simulink model "zad3_sim"  (R2014b)
settings: Solver=ode45  StartTime=0.0  StopTime=70  MaxStep=10  RelTol=1e-3
values from neighbouring files (symbols this model uses):
  a1 = -0.28    [set_params.m]
  a2 = -0.9    [set_params.m]
  a3 = 0.35    [set_params.m]
  a4 = 0.3    [set_params.m]
  K = 4.5    [set_params.m]
  T1 = 5    [set_params.m]
  T2 = 8    [set_params.m]
  Tp = 1    [zad10.m]    (also in zad11.m; zad3.m = Tp_vect(i); zad9.m)
settings Model: Creator=kuba  LastModifiedBy=kuba
settings DebuggingCC: SolverPrmCheckMsg=none

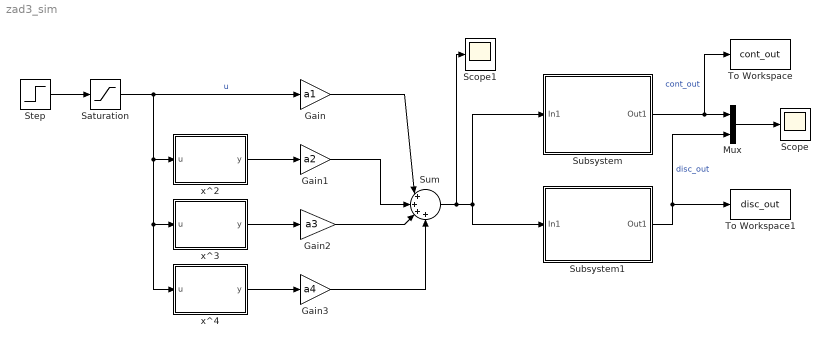
== system zad3_sim ==
  Gain : Gain  Gain=a1
  Gain1 : Gain  Gain=a2
  Gain2 : Gain  Gain=a3
  Gain3 : Gain  Gain=a4
  Mux : Mux  Inputs=2
  Saturation : Saturate  UpperLimit=1  LowerLimit=-1
  Scope : Scope
  Scope1 : Scope
  Step : Step  SampleTime=0
  Subsystem : Subsystem  Tag=Model ciągły  Description=Model ciągły
  Subsystem1 : Subsystem
  Sum : Sum  Inputs=|++++
  To Workspace : ToWorkspace  VariableName=cont_out  SaveFormat=Timeseries  SampleTime=-1
      settings: Save2DSignal=2-D array (concatenate along first dimension)
  To Workspace1 : ToWorkspace  VariableName=disc_out  SaveFormat=Timeseries  SampleTime=-1
  x^2 : MATLAB Function  TreatAsAtomicUnit=on
  x^3 : MATLAB Function  TreatAsAtomicUnit=on
  "x^4 " : MATLAB Function  TreatAsAtomicUnit=on
  wires:
  Saturation/1 -> "x^4 "/1(u), x^3/1(u), x^2/1(u), Gain/1  "u"
  x^2/1(y) -> Gain1/1
  x^3/1(y) -> Gain2/1
  "x^4 "/1(y) -> Gain3/1
  Gain/1 -> Sum/1
  Gain1/1 -> Sum/2
  Gain2/1 -> Sum/3
  Gain3/1 -> Sum/4
  Sum/1 -> Scope1/1, Subsystem1/1(In1), Subsystem/1(In1)
  Subsystem/1(Out1) -> To Workspace/1, Mux/1  "cont_out"
  Subsystem1/1(Out1) -> To Workspace1/1, Mux/2  "disc_out"
  Mux/1 -> Scope/1
  Step/1 -> Saturation/1

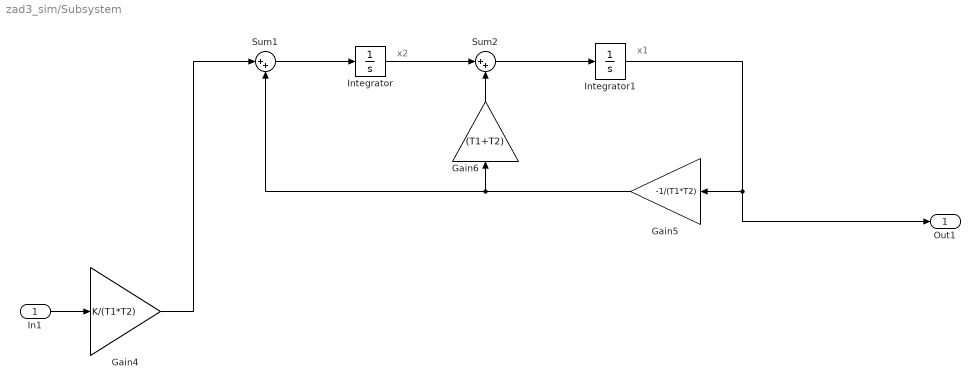
== system zad3_sim/Subsystem ==
  note: x2
  note: x1
  In1 : Inport
  Gain4 : Gain  Gain=K/(T1*T2)
  Gain5 : Gain  Gain=-1/(T1*T2)
  Gain6 : Gain  Gain=(T1+T2)
  Integrator : Integrator
  Integrator1 : Integrator
  Sum1 : Sum  Inputs=|++
  Sum2 : Sum  Inputs=|++
  Out1 : Outport
  wires:
  In1/1 -> Gain4/1
  Sum1/1 -> Integrator/1
  Gain4/1 -> Sum1/1
  Sum2/1 -> Integrator1/1
  Integrator/1 -> Sum2/1
  Integrator1/1 -> Out1/1, Gain5/1
  Gain5/1 -> Gain6/1, Sum1/2
  Gain6/1 -> Sum2/2

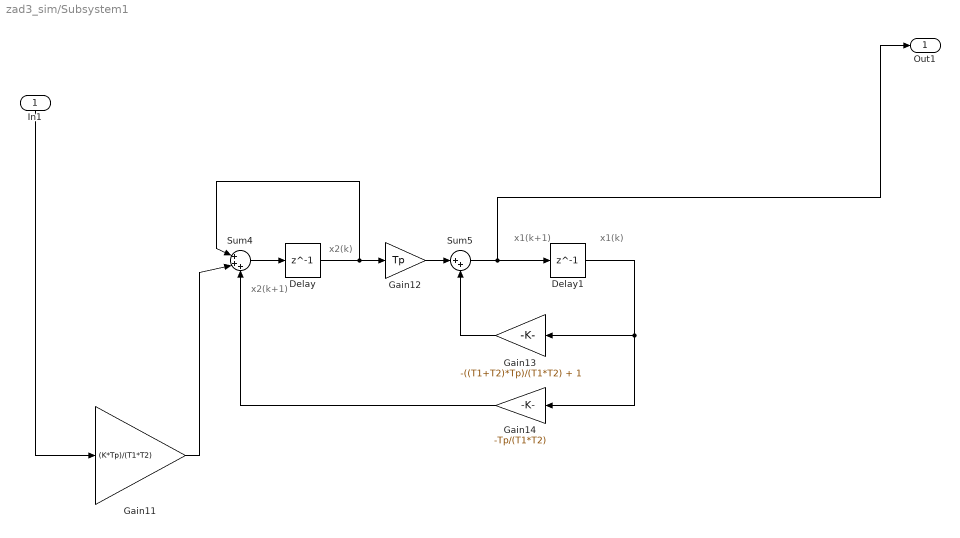
== system zad3_sim/Subsystem1 ==
  note: x2(k+1)
  note: x2(k)
  note: x1(k+1)
  note: x1(k)
  In1 : Inport
  Delay : Delay  DelayLength=1  SampleTime=Tp
  Delay1 : Delay  DelayLength=1  SampleTime=Tp
  Gain11 : Gain  Gain=(K*Tp)/(T1*T2)
  Gain12 : Gain  Gain=Tp
  Gain13 : Gain  Gain=-((T1+T2)*Tp)/(T1*T2) + 1
  Gain14 : Gain  Gain=-Tp/(T1*T2)
  Sum4 : Sum  Inputs=|+++
  Sum5 : Sum  Inputs=|++
  Out1 : Outport
  wires:
  In1/1 -> Gain11/1
  Sum4/1 -> Delay/1
  Gain11/1 -> Sum4/2
  Gain12/1 -> Sum5/1
  Gain13/1 -> Sum5/2
  Delay/1 -> Gain12/1, Sum4/1
  Delay1/1 -> Gain14/1, Gain13/1
  Sum5/1 -> Out1/1, Delay1/1
  Gain14/1 -> Sum4/3

== matlab function zad3_sim/x^3 ==
  data: u input; y output
function y = cube(u)
y = u.^3;

== matlab function zad3_sim/x^2 ==
  data: u input; y output
function y = square(u)
y = u.^2;

== matlab function zad3_sim/x^4  ==
  data: u input; y output
function y = quad(u)
y = u.^4;
